simulink model "MCU_DC_motor"  (R2021b)
settings: Solver=FixedStepAuto  StartTime=0.0  StopTime=10  FixedStep=Ts  RelTol=1e-3
undefined symbols (not defined in the file): B, J, k_e, k_e_hat, k_i, k_is, k_p, k_ps, k_t, L_a, R_a
libraries: simulink x5
settings Model: Creator=YeguKang  LastModifiedBy=qorgud1209
settings SFSimCC: SimCustomInitializer=init_software();  SimUserSources=microcontroller.c
settings SFSimCC: SimCustomHeaderCode=|
  | #include "microcontroller.h"
  | #include "Library/Software/headers/Filters.h"
  | #include "Library/Software/headers/ComplexFilters.h"
  | #include "Constants.h"

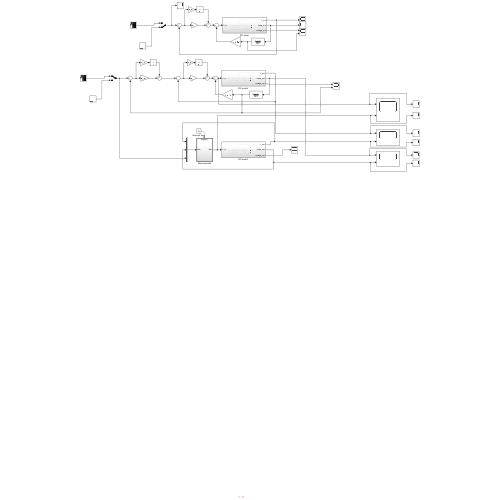
[thumbnail: Simulink's stored preview of the top-level diagram]
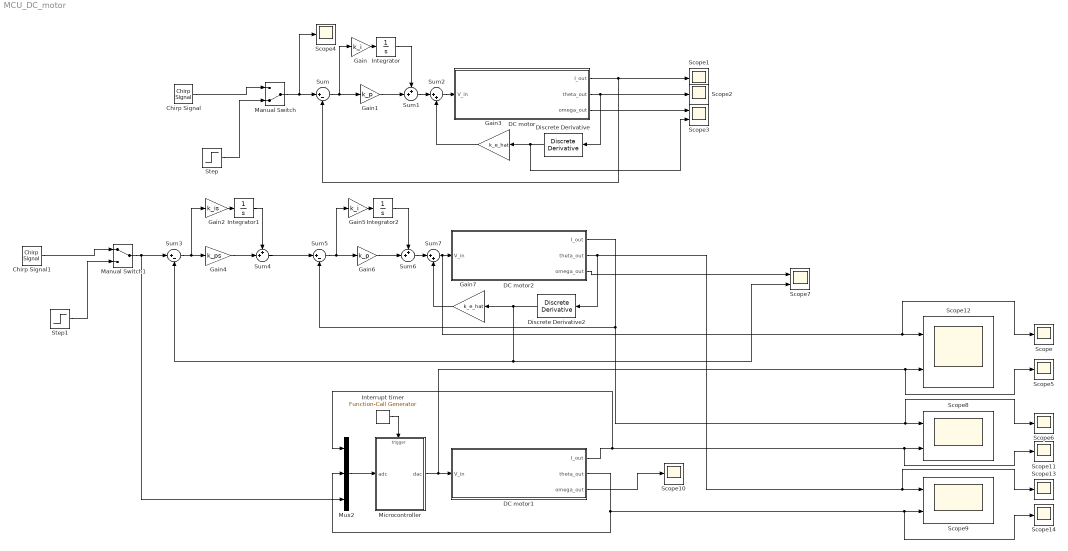
== system MCU_DC_motor ==
  Chirp Signal : simulink/Sources/Chirp Signal  f1=0.1  T=10  f2=300
  Chirp Signal1 : simulink/Sources/Chirp Signal  f1=0.1  T=10  f2=30
  DC motor : Subsystem
  DC motor1 : Subsystem
  DC motor2 : Subsystem
  Discrete Derivative : simulink/Discrete/Discrete Derivative  gainval=1.0  ICPrevScaledInput=0.0  OutMin=[]  OutMax=[]  OutDataType=fixdt(1, 16)  OutScaling=2^-10  DoSatur=off
  Discrete Derivative2 : simulink/Discrete/Discrete Derivative  gainval=1.0  ICPrevScaledInput=0.0  OutMin=[]  OutMax=[]  OutDataType=fixdt(1, 16)  OutScaling=2^-10  DoSatur=off
  Gain : Gain  Gain=k_i
  Gain1 : Gain  Gain=k_p
  Gain2 : Gain  Gain=k_is
  Gain3 : Gain  Gain=k_e_hat
  Gain4 : Gain  Gain=k_ps
  Gain5 : Gain  Gain=k_i
  Gain6 : Gain  Gain=k_p
  Gain7 : Gain  Gain=k_e_hat
  Integrator : Integrator
  Integrator1 : Integrator
  Integrator2 : Integrator
  Interrupt timer : simulink/Ports & Subsystems/Function-Call Generator  sample_time=Ts  numberOfIterations=1  DisallowWideOutput=off
  Manual Switch : ManualSwitch  CurrentSetting=0
  Manual Switch1 : ManualSwitch
  Microcontroller : Subsystem
  Mux2 : Mux  Inputs=[1 1 1]
  Scope{,1..2,4..6,10..11,13..14} (10 alike) : Scope
  Scope{3,7..9,12} (5 alike) : Scope  NumInputPorts=2
  Step : Step  SampleTime=0
  Step1 : Step  SampleTime=0
  Sum : Sum  Inputs=|+-
  Sum1 : Sum  Inputs=++|
  Sum2 : Sum  Inputs=|++
  Sum3 : Sum  Inputs=|+-
  Sum4 : Sum  Inputs=++|
  Sum5 : Sum  Inputs=|+-
  Sum6 : Sum  Inputs=++|
  Sum7 : Sum  Inputs=|++
  wires:
  Interrupt timer/1 -> Microcontroller/Trigger
  Mux2/1 -> Microcontroller/1(adc)
  Microcontroller/1(dac) -> Scope5/1, Scope12/2, DC motor1/1(V_in)
  ? -> ?
  Chirp Signal/1 -> Manual Switch/1
  Gain/1 -> Integrator/1
  DC motor/3(omega_out) -> Scope3/1
  DC motor/1(I_out) -> Sum/2, Scope1/1
  Sum1/1 -> Sum2/1
  DC motor/2(theta_out) -> Scope2/1, Discrete Derivative/1
  Sum/1 -> Gain/1, Gain1/1
  Gain1/1 -> Sum1/2
  Integrator/1 -> Sum1/1
  Sum2/1 -> DC motor/1(V_in)
  Discrete Derivative/1 -> Gain3/1, Scope3/2
  Gain3/1 -> Sum2/2
  Step/1 -> Manual Switch/2
  Manual Switch/1 -> Scope4/1, Sum/1
  DC motor2/1(I_out) -> Scope6/1, Scope8/1, Sum5/2
  Gain4/1 -> Sum4/2
  Gain2/1 -> Integrator1/1
  Sum3/1 -> Gain2/1, Gain4/1
  Integrator1/1 -> Sum4/1
  DC motor2/3(omega_out) -> Scope7/1
  Discrete Derivative2/1 -> Gain7/1, Sum3/2, Scope7/2
  Step1/1 -> Manual Switch1/2
  Chirp Signal1/1 -> Manual Switch1/1
  Sum4/1 -> Sum5/1
  Integrator2/1 -> Sum6/1
  Sum5/1 -> Gain5/1, Gain6/1
  Sum6/1 -> Sum7/1
  Gain7/1 -> Sum7/2
  Gain6/1 -> Sum6/2
  Gain5/1 -> Integrator2/1
  Sum7/1 -> Scope/1, Scope12/1, DC motor2/1(V_in)
  DC motor1/3(omega_out) -> Scope10/1
  DC motor1/2(theta_out) -> Mux2/2, Scope14/1, Scope9/2
  Manual Switch1/1 -> Mux2/3, Sum3/1
  DC motor1/1(I_out) -> Mux2/1, Scope11/1, Scope8/2
  DC motor2/2(theta_out) -> Scope13/1, Scope9/1, Discrete Derivative2/1

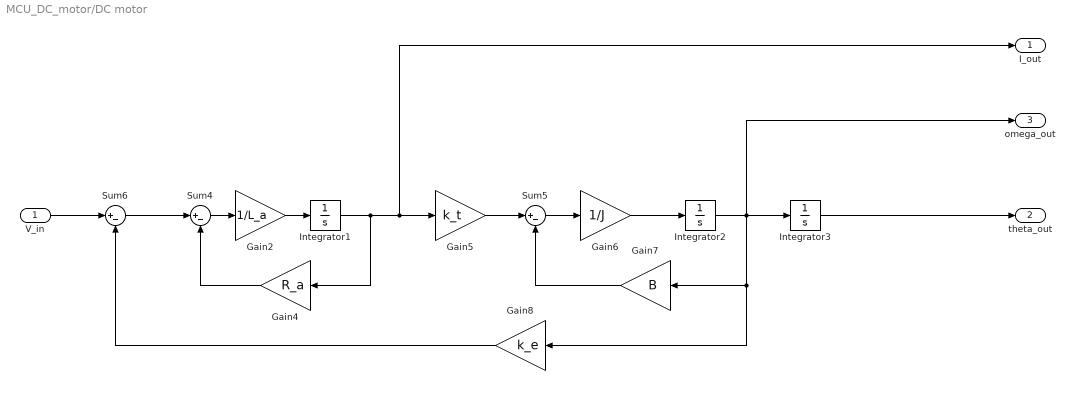
== system MCU_DC_motor/DC motor ==
  V_in : Inport
  Gain2 : Gain  Gain=1/L_a
  Gain4 : Gain  Gain=R_a
  Gain5 : Gain  Gain=k_t
  Gain6 : Gain  Gain=1/J
  Gain7 : Gain  Gain=B
  Gain8 : Gain  Gain=k_e
  Integrator1 : Integrator
  Integrator2 : Integrator
  Integrator3 : Integrator
  Sum4 : Sum  Inputs=|+-
  Sum5 : Sum  Inputs=|+-
  Sum6 : Sum  Inputs=|+-
  I_out : Outport
  theta_out : Outport  Port=2
  omega_out : Outport  Port=3
  wires:
  Integrator2/1 -> omega_out/1, Integrator3/1, Gain7/1, Gain8/1
  Integrator1/1 -> Gain4/1, I_out/1, Gain5/1
  Sum4/1 -> Gain2/1
  Gain4/1 -> Sum4/2
  Gain5/1 -> Sum5/1
  Gain7/1 -> Sum5/2
  Sum6/1 -> Sum4/1
  V_in/1 -> Sum6/1
  Integrator3/1 -> theta_out/1
  Sum5/1 -> Gain6/1
  Gain6/1 -> Integrator2/1
  Gain2/1 -> Integrator1/1
  Gain8/1 -> Sum6/2

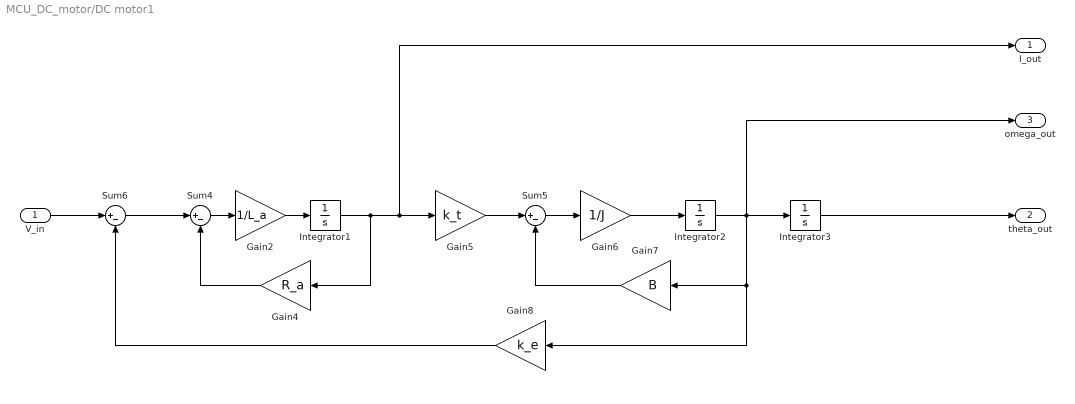
== system MCU_DC_motor/DC motor1 ==
  V_in : Inport
  Gain2 : Gain  Gain=1/L_a
  Gain4 : Gain  Gain=R_a
  Gain5 : Gain  Gain=k_t
  Gain6 : Gain  Gain=1/J
  Gain7 : Gain  Gain=B
  Gain8 : Gain  Gain=k_e
  Integrator1 : Integrator
  Integrator2 : Integrator
  Integrator3 : Integrator
  Sum4 : Sum  Inputs=|+-
  Sum5 : Sum  Inputs=|+-
  Sum6 : Sum  Inputs=|+-
  I_out : Outport
  theta_out : Outport  Port=2
  omega_out : Outport  Port=3
  wires:
  Integrator2/1 -> omega_out/1, Integrator3/1, Gain7/1, Gain8/1
  Integrator1/1 -> Gain4/1, I_out/1, Gain5/1
  Sum4/1 -> Gain2/1
  Gain4/1 -> Sum4/2
  Gain5/1 -> Sum5/1
  Gain7/1 -> Sum5/2
  Sum6/1 -> Sum4/1
  V_in/1 -> Sum6/1
  Integrator3/1 -> theta_out/1
  Sum5/1 -> Gain6/1
  Gain6/1 -> Integrator2/1
  Gain2/1 -> Integrator1/1
  Gain8/1 -> Sum6/2

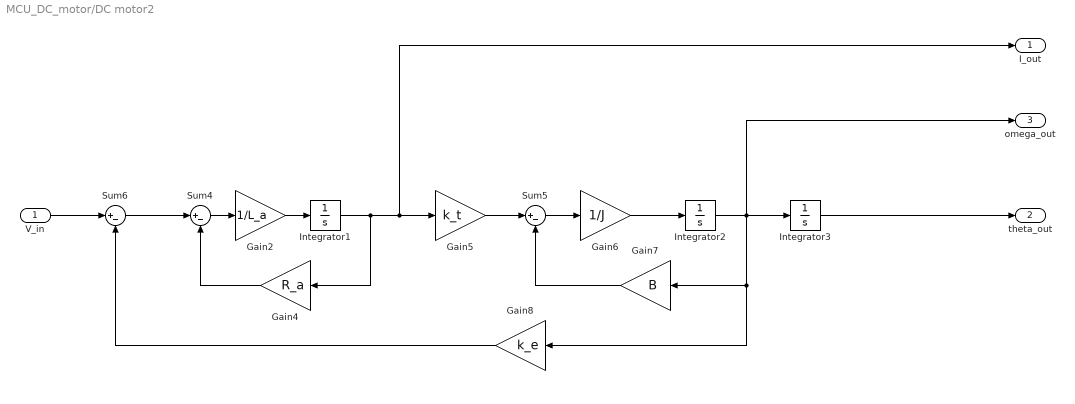
== system MCU_DC_motor/DC motor2 ==
  V_in : Inport
  Gain2 : Gain  Gain=1/L_a
  Gain4 : Gain  Gain=R_a
  Gain5 : Gain  Gain=k_t
  Gain6 : Gain  Gain=1/J
  Gain7 : Gain  Gain=B
  Gain8 : Gain  Gain=k_e
  Integrator1 : Integrator
  Integrator2 : Integrator
  Integrator3 : Integrator
  Sum4 : Sum  Inputs=|+-
  Sum5 : Sum  Inputs=|+-
  Sum6 : Sum  Inputs=|+-
  I_out : Outport
  theta_out : Outport  Port=2
  omega_out : Outport  Port=3
  wires:
  Integrator2/1 -> omega_out/1, Integrator3/1, Gain7/1, Gain8/1
  Integrator1/1 -> Gain4/1, I_out/1, Gain5/1
  Sum4/1 -> Gain2/1
  Gain4/1 -> Sum4/2
  Gain5/1 -> Sum5/1
  Gain7/1 -> Sum5/2
  Sum6/1 -> Sum4/1
  V_in/1 -> Sum6/1
  Integrator3/1 -> theta_out/1
  Sum5/1 -> Gain6/1
  Gain6/1 -> Integrator2/1
  Gain2/1 -> Integrator1/1
  Gain8/1 -> Sum6/2

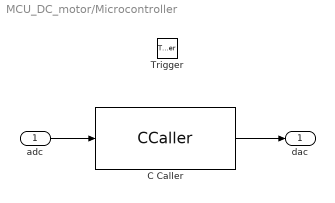
== system MCU_DC_motor/Microcontroller ==
  adc : Inport
  Trigger : TriggerPort  TriggerType=function-call  VariantControl=Variant
  C Caller : CCaller  FunctionName=microcontroller  PortSpecificationStruct="%)30     .    N ,   8    (     @         %    \"     (    !     0         %  0 \"0    $    _    07)G3F%M90  4&]R=$YA;64 4V-O<&4     26YD97@     5'EP90      4VEZ90      27-';&]B86P   X    P    !@    @    $          4    (     0    ,    !         !   P!A9&, #@   #     &    \"     0         !0    @    !     P    $         $  # &%D8P .    .     8    (    !          %    \"     $    %     0         0    !0   $EN<'5T    #@   #@    &    \"     8         !0    @    !     0    $         \"0    @               X    X    !@    @    $          4    (     0    8    !         !     &    9&]U8FQE   .    ,     8    (    !          %    \"     $    !     0         0  $ ,P    X    P    !@    @    ) @        4    (     0    $    !          (  0      #@   #     &    \"     0         !0    @    !     P    $         $  # &1A8P .    ,     8    (    !          %    \"     $    #     0         0  , 9&%C  X    X    !@    @    $          4    (     0    8    !         !     &    3W5T<'5T   .    .     8    (    !@         %    \"     $    !     0         )    \"               #@   #@    &    \"     0         !0    @    !    !@    $         $     8   !D;W5B;&4   X    P    !@    @    $          4    (     0    $    !         !   0 Q    #@   #     &    \"     D\"        !0    @    !     0    $          @ !"
  dac : Outport  VectorParamsAs1DForOutWhenUnconnected=off
  wires:
  C Caller/1 -> dac/1
  adc/1 -> C Caller/1
